simulink model "DPSK_mod"  (R2024a)
settings: Solver=VariableStepAuto  StartTime=0.0  StopTime=10.0  RelTol=1e-3
libraries: simulink x1

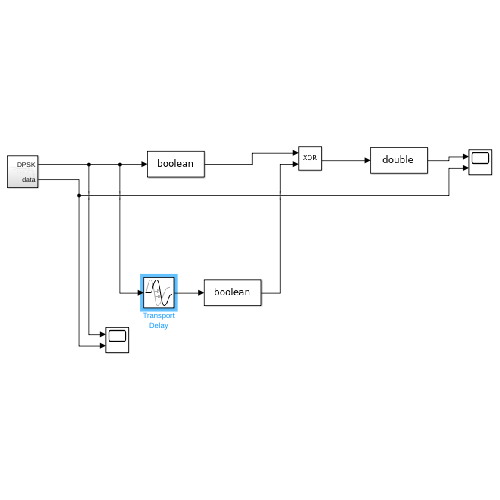
[thumbnail: Simulink's stored preview of the top-level diagram]
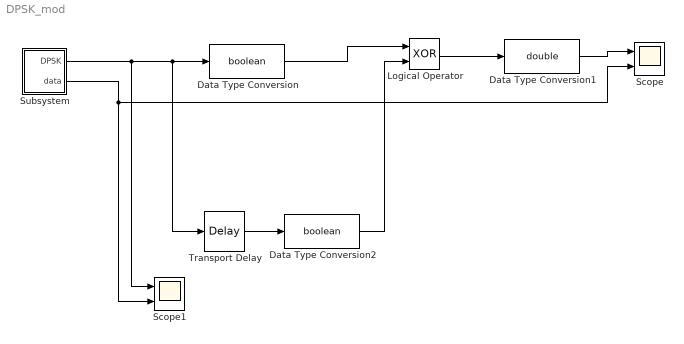
== system DPSK_mod ==
  Data Type Conversion : DataTypeConversion  OutDataTypeStr=boolean  SaturateOnIntegerOverflow=off  RndMeth=Floor
  Data Type Conversion1 : DataTypeConversion  OutDataTypeStr=double  SaturateOnIntegerOverflow=off  RndMeth=Floor
  Data Type Conversion2 : DataTypeConversion  OutDataTypeStr=boolean  SaturateOnIntegerOverflow=off  RndMeth=Floor
  Logical Operator : Logic  Operator=XOR  AllPortsSameDT=off  OutDataTypeStr=boolean
  Scope : Scope  NumInputPorts=2
  Scope1 : Scope  NumInputPorts=2
  Subsystem : Subsystem
  Transport Delay : TransportDelay
  wires:
  Subsystem/1(DPSK) -> Scope1/1, Transport Delay/1, Data Type Conversion/1
  Data Type Conversion/1 -> Logical Operator/1
  Transport Delay/1 -> Data Type Conversion2/1
  Data Type Conversion2/1 -> Logical Operator/2
  Logical Operator/1 -> Data Type Conversion1/1
  Data Type Conversion1/1 -> Scope/1
  Subsystem/2(data) -> Scope1/2, Scope/2

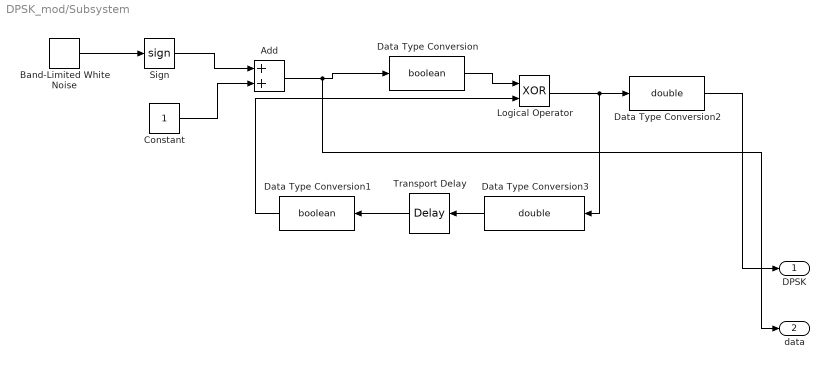
== system DPSK_mod/Subsystem ==
  Add : Sum
  Band-Limited White Noise : simulink/Sources/Band-Limited White Noise  Cov=[0.1]  Ts=0.1  seed=[23341]
  Constant : Constant
  Data Type Conversion : DataTypeConversion  OutDataTypeStr=boolean  SaturateOnIntegerOverflow=off  RndMeth=Floor
  Data Type Conversion1 : DataTypeConversion  OutDataTypeStr=boolean  SaturateOnIntegerOverflow=off  RndMeth=Floor
  Data Type Conversion2 : DataTypeConversion  OutDataTypeStr=double  SaturateOnIntegerOverflow=off  RndMeth=Floor
  Data Type Conversion3 : DataTypeConversion  OutDataTypeStr=double  SaturateOnIntegerOverflow=off  RndMeth=Floor
  Logical Operator : Logic  Operator=XOR  AllPortsSameDT=off  OutDataTypeStr=boolean
  Sign : Signum
  Transport Delay : TransportDelay  DelayTime=0
  DPSK : Outport
  data : Outport  Port=2
  wires:
  Band-Limited White Noise/1 -> Sign/1
  Constant/1 -> Add/2
  Data Type Conversion1/1 -> Logical Operator/2
  Data Type Conversion2/1 -> DPSK/1
  Data Type Conversion/1 -> Logical Operator/1
  Add/1 -> data/1, Data Type Conversion/1
  Transport Delay/1 -> Data Type Conversion1/1
  Data Type Conversion3/1 -> Transport Delay/1
  Sign/1 -> Add/1
  Logical Operator/1 -> Data Type Conversion2/1, Data Type Conversion3/1
